simulink model "dc_motor"  (R2020b)
settings: Solver=VariableStepAuto  StartTime=0.0  StopTime=0.1  RelTol=1e-3
undefined symbols (not defined in the file): b, I, J, k_tau, R
settings Model: Creator=casla195  LastModifiedBy=Casper
settings SFSimCC: CustomCodeUndefinedFunction=UseInterfaceOnly

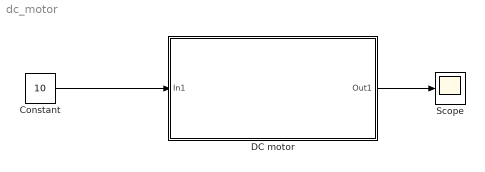
== system dc_motor ==
  Constant : Constant  Value=10
  "DC motor " : Subsystem
  Scope : Scope
  wires:
  Constant/1 -> "DC motor "/1(In1)
  "DC motor "/1(Out1) -> Scope/1

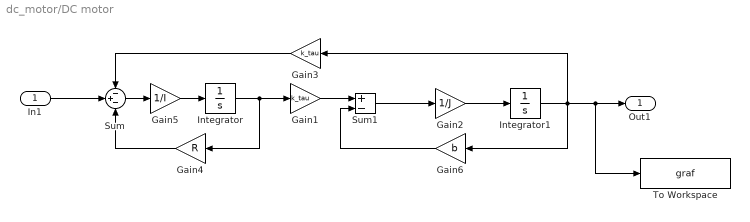
== system dc_motor/DC motor  ==
  In1 : Inport
  Gain1 : Gain  Gain=k_tau
  Gain2 : Gain  Gain=1/J
  Gain3 : Gain  Gain=k_tau
  Gain4 : Gain  Gain=R
  Gain5 : Gain  Gain=1/I
  Gain6 : Gain  Gain=b
  Integrator : Integrator
  Integrator1 : Integrator
  Sum : Sum  Inputs=-+-
  Sum1 : Sum  Inputs=+-
  To Workspace : ToWorkspace  VariableName=graf  SaveFormat=Timeseries  SampleTime=-1
  Out1 : Outport  VectorParamsAs1DForOutWhenUnconnected=off
  wires:
  Integrator/1 -> Gain4/1, Gain1/1
  Gain3/1 -> Sum/1
  Sum/1 -> Gain5/1
  Gain4/1 -> Sum/3
  Sum1/1 -> Gain2/1
  Gain5/1 -> Integrator/1
  Integrator1/1 -> Gain6/1, Gain3/1, To Workspace/1, Out1/1
  Gain2/1 -> Integrator1/1
  Gain6/1 -> Sum1/2
  Gain1/1 -> Sum1/1
  In1/1 -> Sum/2
